simulink model "PumpSeries_linearOrQuadraticCharacter"  (R2018b)
settings: Solver=ode45  StartTime=0.0  StopTime=100  MaxStep=5  RelTol=1e-3  EnableMultiTasking=on
undefined symbols (not defined in the file): DiameterLastPiece, DPConstant, DPLinear, DPQuadratic, ID, MassFlow, path_carnot, Pressure, Temperature, Water
libraries: carnot x15, simulink x3
settings Model: EnablePacing=on  Creator=drhf  LastModifiedBy=drhf
settings DataIOCC: SaveFormat=Array  SignalLoggingSaveFormat=ModelDataLogs
settings OptimizationCC: ExpressionDepthLimit=2147483647  LifeSpan=inf
settings DebuggingCC: UnderspecifiedInitializationDetection=Classic  MergeDetectMultiDrivingBlocksExec=none  SolverPrmCheckMsg=warning  StateNameClashWarn=warning  SFUnexpectedBacktrackingDiag=warning  SFNoUnconditionalDefaultTransitionDiag=warning  SFExecutionAtInitializationDiag=none
settings HardwareCC: ProdBitPerPointer=32  ProdBitPerSizeT=32  ProdBitPerPtrDiffT=32  ProdLargestAtomicFloat=None  ProdIntDivRoundTo=Undefined  ProdEndianess=Unspecified  ProdWordSize=32  ProdHWDeviceType=32-bit Generic
settings ModelReferenceCC: PropagateSignalLabelsOutOfModel=off
settings SFSimCC: SimUseLocalCustomCode=off
settings RTWCC: RTWUseLocalCustomCode=off
settings CodeAppCC: StateflowObjectComments=on
settings GRTTargetCC: TargetLangStandard=C89/C90 (ANSI)  GeneratePreprocessorConditionals=Disable all  CombineOutputUpdateFcns=off  GRTInterface=on
settings ConfigComp: CovMetricSettings=dw  CovHtmlReporting=on  CovSaveCumulativeToWorkspaceVar=on  CovSaveSingleToWorkspaceVar=on  CovExternalEMLEnable=off

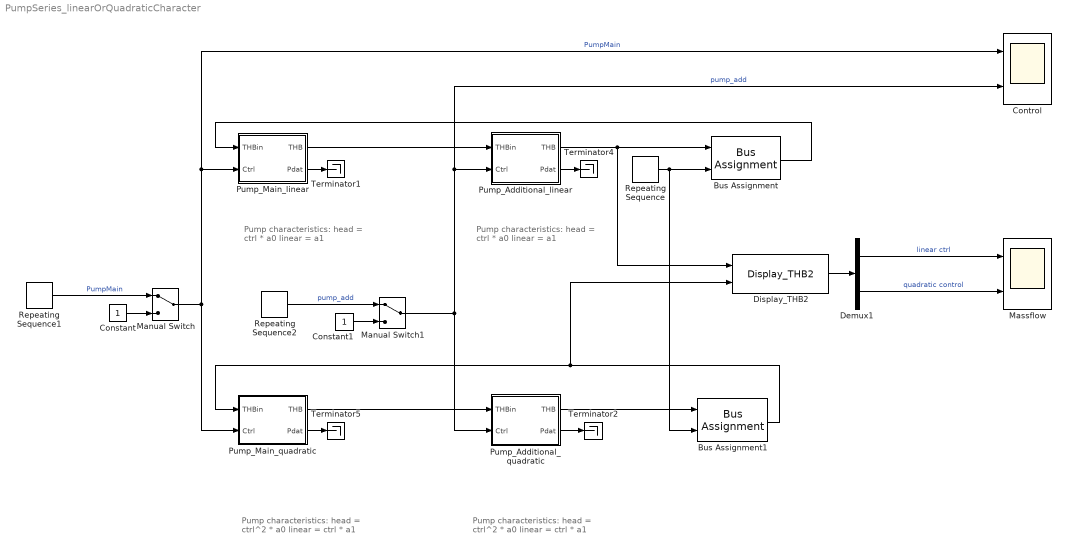
== system PumpSeries_linearOrQuadraticCharacter ==
  note: Pump characteristics:
      | head = ctrl^2 * a0
      | linear = ctrl * a1
  note: Pump characteristics:
      | head = ctrl * a0
      | linear = a1
  note: Pump characteristics:
      | head = ctrl * a0
      | linear = a1
  note: Pump characteristics:
      | head = ctrl^2 * a0
      | linear = ctrl * a1
  Bus Assignment : BusAssignment  AssignedSignals=DPQuadratic
  Bus Assignment1 : BusAssignment  AssignedSignals=DPQuadratic
  Constant : Constant
  Constant1 : Constant
  Control : Scope  NumInputPorts=2
  Demux1 : Demux  Outputs=2
  Display_THB2 : carnot/Outputs/Display_THB2  t=off  m=on  p=off  id=off  mix=off  d=off
      settings: SourceProductName=Carnot
  Manual Switch : ManualSwitch
  Manual Switch1 : ManualSwitch
  Massflow : Scope  NumInputPorts=2
  Pump_Additional_linear : Subsystem  AncestorBlock=carnot/Hydraulics/Pump_Additional  mask(Pump Additional){Tini=20, PathName=fullfile(path_carnot('libsl'), 'Hydraulics', 'Pump_Main', 'parameter_set'), FileName='Pump6m.mat', userPath=off, userParam=off, a0=60000, a1=-43200, a2=0, dia=0.025, UA=1, mcp=4182, e0=50, e1=28.8, e2=-10.368}
      mask prompts: Tini "Ambient temperature for losses and initial temperture in °C"; PathName "Path"; FileName "Parameter set"; userPath "Edit path and name of parameter set"; userParam "User defined parameters"; a0 "a0: pump head in [Pa] (pressure increase at zero flow)"; a1 "a1: pump characteristic linear coefficient [Pa*s/kg]"; a2 "a2: pump characteristic quadratic coefficient [Pa*(s/kg)²]"; dia "Diameter at in- and outlet [m]"; UA "UA: thermal loss coefficient in W/K"; mcp "mcp: thermal capacity of the node in J/K"; e0 "e0: constant coefficient in W"; e1 "e1: linear coefficient in W*s/kg"; e2 "e2: quadratic coefficient in W*(s/kg)²"
      mask help:
      | This is an additional pump in a circuit. Every circuit must have exactly ONE 'Pump_Main'. It may have several 'Pump_Additional' blocks. The pump adds pump_head to the pressure drop of the circuit dp_circuit:
      |     dp_circuit = c + l*mdot + q*(mdot)²
      |     pump_head_ = a0*Ctrl² + a1*Ctrl*mdot +a2*mdot²
      |     dp_total = pump_head - dp_circuit
      |     p1 = system_pressure + (a0*Ctrl² - c) + (a1*Ctrl - l) * mdot + (a2-q)*(mdot)²
      | with
      |   Ctrl : Control signal input [0..1]
      | Note: Pump_Additional uses the parameters sets as Pump_Main.
      mask init:
      | % callback to set parameters of model
      | [ok, param] = CarnotCallbacks_PumpAdditional('SetParameters',gcbh,PathName,FileName);
      mask Help: web(fullfile(path_carnot('help'),'Pump_Main.html'),'-helpbrowser')
      mask TypeOptions Tini: ThermalNodeTHB/Tini
      mask Callback userPath: [ok, param] = CarnotCallbacks_PumpAdditional('UserEdit',gcbh);
      mask Callback userParam: [ok, param] = CarnotCallbacks_PumpAdditional('UserEdit',gcbh);
      mask TypeOptions a0: PumpHead/Gain
      mask TypeOptions a1: PumpLinear/Gain
      mask TypeOptions a2: PumpQuadratic/Value
      mask TypeOptions dia: dia/Value
      mask TypeOptions UA: ThermalNodeTHB/UA
      mask TypeOptions mcp: ThermalNodeTHB/mcp
      mask TypeOptions e0: ElectricConsumptionPump/e0
      mask TypeOptions e1: ElectricConsumptionPump/e1
      mask TypeOptions e2: ElectricConsumptionPump/e2
      mask DialogControl ParameterGroupFile Prompt: Picking a parameter set
      mask DialogControl Control1 Prompt: Carnot public data
      mask DialogControl Control1 Callback: [ok, file] = CarnotCallbacks_PumpAdditional('GetFilename',gcbh,'public');
      mask DialogControl Control3 Prompt: Carnot internal data
      mask DialogControl Control3 Callback: [ok, file] = CarnotCallbacks_PumpAdditional('GetFilename',gcbh,'internal');
      mask DialogControl Control4 Prompt: Selected path
      mask DialogControl Control4 Callback: [ok, file] = CarnotCallbacks_PumpAdditional('GetFilename',gcbh,'selected');
      mask DialogControl PrameterGroupUser Prompt: Parameter Values
      mask DialogControl Container9 Prompt: Hydraulic
      mask DialogControl Container7 Prompt: Thermal
      mask DialogControl Control9 Prompt: Thermal node for temperature:  mcp * dTnode/dt = UA*(Tamb-Tnode) + mdot*cp_in*(Tin-Tnode)
      mask DialogControl Container12 Prompt: Electric
      mask DialogControl Control7 Prompt: Power consumption  Pel = e0 + e1*mdot + e2*mdot²
      mask DialogControl Control5 Prompt: Save in Carnot internal data
      mask DialogControl Control5 Callback: [ok, param] = CarnotCallbacks_PumpAdditional('SaveFilename',gcbh,'internal','B');
      mask DialogControl Control6 Prompt: Save in selected path
      mask DialogControl Control6 Callback: [ok, param] = CarnotCallbacks_PumpAdditional('SaveFilename',gcbh,'selected','B');
      mask Display:
      | % user defined picture file
      | picfile = fullfile(path_carnot('intlibsl'), ...
      |         'Hydraulics', 'Pump_Additional', 'PumpAdditional.jpg');
      | 
      | pic = false;
      | if ~BlockIsInCarnotLibrary    % if not located in library any more
      |     if exist(picfile,'file') % show internal picture if defined
      |         image(imread(picfile), [0.2, 0, 0.6, 1])
      |         set_param(gcb, 'BackgroundColor', 'White')
      |         pic = true;
      |     end
      | end
      | if ~pic    % show public picture
      |     set_param(gcb, 'BackgroundColor', 'green')
      |     plot(0,0,1,1,[40,70,40,30,30,40,60,70,70,60,40]/100, ...
      |         [70,50,30,40,60,70,70,60,40,30,30]/100)
      |     disp('add')
      | end
  Pump_Additional_quadratic : Subsystem  AncestorBlock=carnot/Hydraulics/Pump_Additional  mask(Pump Additional){Tini=20, PathName=fullfile(path_carnot('libsl'), 'Hydraulics', 'Pump_Main', 'parameter_set'), FileName='Pump6m.mat', userPath=off, userParam=off, a0=60000, a1=-43200, a2=0, dia=0.025, UA=1, mcp=4182, e0=50, e1=28.8, e2=-10.368}
      mask prompts: Tini "Ambient temperature for losses and initial temperture in °C"; PathName "Path"; FileName "Parameter set"; userPath "Edit path and name of parameter set"; userParam "User defined parameters"; a0 "a0: pump head in [Pa] (pressure increase at zero flow)"; a1 "a1: pump characteristic linear coefficient [Pa*s/kg]"; a2 "a2: pump characteristic quadratic coefficient [Pa*(s/kg)²]"; dia "Diameter at in- and outlet [m]"; UA "UA: thermal loss coefficient in W/K"; mcp "mcp: thermal capacity of the node in J/K"; e0 "e0: constant coefficient in W"; e1 "e1: linear coefficient in W*s/kg"; e2 "e2: quadratic coefficient in W*(s/kg)²"
      mask help:
      | This is an additional pump in a circuit. Every circuit must have exactly ONE 'Pump_Main'. It may have several 'Pump_Additional' blocks. The pump adds pump_head to the pressure drop of the circuit dp_circuit:
      |     dp_circuit = c + l*mdot + q*(mdot)²
      |     pump_head_ = a0*Ctrl² + a1*Ctrl*mdot +a2*mdot²
      |     dp_total = pump_head - dp_circuit
      |     p1 = system_pressure + (a0*Ctrl² - c) + (a1*Ctrl - l) * mdot + (a2-q)*(mdot)²
      | with
      |   Ctrl : Control signal input [0..1]
      | Note: Pump_Additional uses the parameters sets as Pump_Main.
      mask init:
      | % callback to set parameters of model
      | [ok, param] = CarnotCallbacks_PumpAdditional('SetParameters',gcbh,PathName,FileName);
      mask Help: web(fullfile(path_carnot('help'),'Pump_Main.html'),'-helpbrowser')
      mask TypeOptions Tini: ThermalNodeTHB/Tini
      mask Callback userPath: [ok, param] = CarnotCallbacks_PumpAdditional('UserEdit',gcbh);
      mask Callback userParam: [ok, param] = CarnotCallbacks_PumpAdditional('UserEdit',gcbh);
      mask TypeOptions a0: PumpHead/Gain
      mask TypeOptions a1: PumpLinear/Gain
      mask TypeOptions a2: PumpQuadratic/Value
      mask TypeOptions dia: dia/Value
      mask TypeOptions UA: ThermalNodeTHB/UA
      mask TypeOptions mcp: ThermalNodeTHB/mcp
      mask TypeOptions e0: ElectricConsumptionPump/e0
      mask TypeOptions e1: ElectricConsumptionPump/e1
      mask TypeOptions e2: ElectricConsumptionPump/e2
      mask DialogControl ParameterGroupFile Prompt: Picking a parameter set
      mask DialogControl Control1 Prompt: Carnot public data
      mask DialogControl Control1 Callback: [ok, file] = CarnotCallbacks_PumpAdditional('GetFilename',gcbh,'public');
      mask DialogControl Control3 Prompt: Carnot internal data
      mask DialogControl Control3 Callback: [ok, file] = CarnotCallbacks_PumpAdditional('GetFilename',gcbh,'internal');
      mask DialogControl Control4 Prompt: Selected path
      mask DialogControl Control4 Callback: [ok, file] = CarnotCallbacks_PumpAdditional('GetFilename',gcbh,'selected');
      mask DialogControl PrameterGroupUser Prompt: Parameter Values
      mask DialogControl Container9 Prompt: Hydraulic
      mask DialogControl Container7 Prompt: Thermal
      mask DialogControl Control9 Prompt: Thermal node for temperature:  mcp * dTnode/dt = UA*(Tamb-Tnode) + mdot*cp_in*(Tin-Tnode)
      mask DialogControl Container12 Prompt: Electric
      mask DialogControl Control7 Prompt: Power consumption  Pel = e0 + e1*mdot + e2*mdot²
      mask DialogControl Control5 Prompt: Save in Carnot internal data
      mask DialogControl Control5 Callback: [ok, param] = CarnotCallbacks_PumpAdditional('SaveFilename',gcbh,'internal','B');
      mask DialogControl Control6 Prompt: Save in selected path
      mask DialogControl Control6 Callback: [ok, param] = CarnotCallbacks_PumpAdditional('SaveFilename',gcbh,'selected','B');
      mask Display:
      | % user defined picture file
      | picfile = fullfile(path_carnot('intlibsl'), ...
      |         'Hydraulics', 'Pump_Additional', 'PumpAdditional.jpg');
      | 
      | pic = false;
      | if ~BlockIsInCarnotLibrary    % if not located in library any more
      |     if exist(picfile,'file') % show internal picture if defined
      |         image(imread(picfile), [0.2, 0, 0.6, 1])
      |         set_param(gcb, 'BackgroundColor', 'White')
      |         pic = true;
      |     end
      | end
      | if ~pic    % show public picture
      |     set_param(gcb, 'BackgroundColor', 'green')
      |     plot(0,0,1,1,[40,70,40,30,30,40,60,70,70,60,40]/100, ...
      |         [70,50,30,40,60,70,70,60,40,30,30]/100)
      |     disp('add')
      | end
  Pump_Main_linear : Subsystem  AncestorBlock=carnot/Hydraulics/Pump_Main  mask(Pump Main){Tini=20, p0=3e5, IDpreset=pressure drop, fluid=Water, mix=0, mix2=0, mix3=0, t1=1, PathName=fullfile(path_carnot('libsl'), 'Hydraulics', 'Pump_Main', 'parameter_set'), FileName='Pump6m.mat', userPath=off, userParam=off, a0=60000, a1=-43200, a2=0, dia=0.025, UA=1, mcp=4182, e0=50, e1=28.8, e2=-10.368}
      mask prompts: Tini "Ambient temperature for losses and initial temperture in °C"; p0 "System pressure at pump inlet [Pa]"; IDpreset "Pressure calculation"; mix "Fluid mixture    [0..1]"; mix2 "Fluid mixture 2 [0..1]"; mix3 "Fluid mixture 3 [0..1]"; t1 "Time constant [s] of pump"; PathName "Path"; FileName "Parameter set"; userPath "Edit path and name of parameter set"; userParam "User defined parameters"; a0 "a0: pump head in [Pa] (pressure increase at zero flow)"; a1 "a1: pump characteristic linear coefficient [Pa*s/kg]"; a2 "a2: pump characteristic quadratic coefficient [Pa*(s/kg)²]"; dia "Diameter at in- and outlet [m]"; UA "UA: thermal loss coefficient in W/K"; mcp "mcp: thermal capacity of the node in J/K"; e0 "e0: constant coefficient in W"; e1 "e1: linear coefficient in W*s/kg"; e2 "e2: quadratic coefficient in W*(s/kg)²"
      mask help:
      | This is the main pump in a circuit. Every circuit must have exactly ONE 'Pump_Main'. Use the 'Pump_Additional' blocks if you want to use more pumps.
      | The Pump_Main calculate massflow by setting pressure drop in the circuit (dp_circuit) equal to the pressure increase of the pump (pump_head).
      |   dp_circuit = c + l*mdot + q*mdot²
      |   pump_head_ = a0*Ctrl² + a1*Ctrl*mdot +a2*mdot²
      | with
      |   mdot : massflow in kg/s
      |   Ctrl : Control signal input [0..1]
      | This model uses a Memory block to break an algebraic loop. Avoid using the variable-step solver ode15s or ode113 (see block help for details).
      | A unit delay block with a sample time ("time constant of the pump") limits the maximum stepsize.
      mask init:
      | % callback to set parameters of model
      | [ok, param] = CarnotCallbacks_PumpMain('SetParameters',gcbh,PathName,FileName);
      mask Help: web(fullfile(path_carnot('help'),'Pump_Main.html'),'-helpbrowser')
      mask TypeOptions Tini: ThermalNodeTHB/Tini
      mask TypeOptions p0: basic_THB/p
      mask TypeOptions IDpreset: ID/IDpreset
      mask TypeOptions fluid: basic_THB/fluid
      mask TypeOptions mix: basic_THB/mix
      mask TypeOptions mix2: basic_THB/mix2
      mask TypeOptions mix3: basic_THB/mix3
      mask TypeOptions t1: UnitDelay/SampleTime
      mask Callback userPath: [ok, param] = CarnotCallbacks_PumpMain('UserEdit',gcbh);
      mask Callback userParam: [ok, param] = CarnotCallbacks_PumpMain('UserEdit',gcbh);
      mask TypeOptions a0: PumpHead/Gain
      mask TypeOptions a1: PumpLinear/Value
      mask TypeOptions a2: PumpQuadratic/Value
      mask TypeOptions dia: basic_THB/dia
      mask TypeOptions UA: ThermalNodeTHB/UA
      mask TypeOptions mcp: ThermalNodeTHB/mcp
      mask TypeOptions e0: ElectricConsumptionPump/e0
      mask TypeOptions e1: ElectricConsumptionPump/e1
      mask TypeOptions e2: ElectricConsumptionPump/e2
      mask DialogControl ParameterGroupFile Prompt: Picking a parameter set
      mask DialogControl Control1 Prompt: Carnot public data
      mask DialogControl Control1 Callback: [ok, file] = CarnotCallbacks_PumpMain('GetFilename',gcbh,'public');
      mask DialogControl Control3 Prompt: Carnot internal data
      mask DialogControl Control3 Callback: [ok, file] = CarnotCallbacks_PumpMain('GetFilename',gcbh,'internal');
      mask DialogControl Control4 Prompt: Selected path
      mask DialogControl Control4 Callback: [ok, file] = CarnotCallbacks_PumpMain('GetFilename',gcbh,'selected');
      mask DialogControl PrameterGroupUser Prompt: Parameter Values
      mask DialogControl Container9 Prompt: Hydraulic
      mask DialogControl Container7 Prompt: Thermal
      mask DialogControl Control9 Prompt: Thermal node for temperature:  mcp * dTnode/dt = UA*(Tamb-Tnode) + mdot*cp_in*(Tin-Tnode)
      mask DialogControl Container14 Prompt: Electric
      mask DialogControl Control7 Prompt: Power consumption  Pel = e0 + e1*mdot + e2*mdot²
      mask DialogControl Control5 Prompt: Save in Carnot internal data
      mask DialogControl Control5 Callback: [ok, param] = CarnotCallbacks_PumpMain('SaveFilename',gcbh,'internal','B');
      mask DialogControl Control6 Prompt: Save in selected path
      mask DialogControl Control6 Callback: [ok, param] = CarnotCallbacks_PumpMain('SaveFilename',gcbh,'selected','B');
      mask Display:
      | % user defined picture file
      | picfile = fullfile(path_carnot('intlibsl'), ...
      |         'Hydraulics', 'Pump_Main', 'PumpMain.jpg');
      | 
      | pic = false;
      | if ~BlockIsInCarnotLibrary    % if not located in library any more
      |     if exist(picfile,'file') % show internal picture if defined
      |         image(imread(picfile), [0.2, 0, 0.6, 1])
      |         set_param(gcb, 'BackgroundColor', 'White')
      |         pic = true;
      |     end
      | end
      | if ~pic    % show public picture
      |     set_param(gcb, 'BackgroundColor', 'green')
      |     plot(0,0,1,1,[40,70,40,30,30,40,60,70,70,60,40]/100, ...
      |         [70,50,30,40,60,70,70,60,40,30,30]/100)
      |     disp('main')
      | end
  Pump_Main_quadratic : Subsystem  AncestorBlock=carnot/Hydraulics/Pump_Main  mask(Pump Main){Tini=20, p0=3e5, IDpreset=pressure drop, fluid=Water, mix=0, mix2=0, mix3=0, t1=1, PathName=fullfile(path_carnot('libsl'), 'Hydraulics', 'Pump_Main', 'parameter_set'), FileName='Pump6m.mat', userPath=off, userParam=off, a0=60000, a1=-43200, a2=0, dia=0.025, UA=1, mcp=4182, e0=50, e1=28.8, e2=-10.368}
      mask prompts: Tini "Ambient temperature for losses and initial temperture in °C"; p0 "System pressure at pump inlet [Pa]"; IDpreset "Pressure calculation"; mix "Fluid mixture    [0..1]"; mix2 "Fluid mixture 2 [0..1]"; mix3 "Fluid mixture 3 [0..1]"; t1 "Time constant [s] of pump"; PathName "Path"; FileName "Parameter set"; userPath "Edit path and name of parameter set"; userParam "User defined parameters"; a0 "a0: pump head in [Pa] (pressure increase at zero flow)"; a1 "a1: pump characteristic linear coefficient [Pa*s/kg]"; a2 "a2: pump characteristic quadratic coefficient [Pa*(s/kg)²]"; dia "Diameter at in- and outlet [m]"; UA "UA: thermal loss coefficient in W/K"; mcp "mcp: thermal capacity of the node in J/K"; e0 "e0: constant coefficient in W"; e1 "e1: linear coefficient in W*s/kg"; e2 "e2: quadratic coefficient in W*(s/kg)²"
      mask help:
      | This is the main pump in a circuit. Every circuit must have exactly ONE 'Pump_Main'. Use the 'Pump_Additional' blocks if you want to use more pumps.
      | The Pump_Main calculate massflow by setting pressure drop in the circuit (dp_circuit) equal to the pressure increase of the pump (pump_head).
      |   dp_circuit = c + l*mdot + q*mdot²
      |   pump_head_ = a0*Ctrl² + a1*Ctrl*mdot +a2*mdot²
      | with
      |   mdot : massflow in kg/s
      |   Ctrl : Control signal input [0..1]
      | This model uses a Memory block to break an algebraic loop. Avoid using the variable-step solver ode15s or ode113 (see block help for details).
      | A unit delay block with a sample time ("time constant of the pump") limits the maximum stepsize.
      mask init:
      | % callback to set parameters of model
      | [ok, param] = CarnotCallbacks_PumpMain('SetParameters',gcbh,PathName,FileName);
      mask Help: web(fullfile(path_carnot('help'),'Pump_Main.html'),'-helpbrowser')
      mask TypeOptions Tini: ThermalNodeTHB/Tini
      mask TypeOptions p0: basic_THB/p
      mask TypeOptions IDpreset: ID/IDpreset
      mask TypeOptions fluid: basic_THB/fluid
      mask TypeOptions mix: basic_THB/mix
      mask TypeOptions mix2: basic_THB/mix2
      mask TypeOptions mix3: basic_THB/mix3
      mask TypeOptions t1: UnitDelay/SampleTime
      mask Callback userPath: [ok, param] = CarnotCallbacks_PumpMain('UserEdit',gcbh);
      mask Callback userParam: [ok, param] = CarnotCallbacks_PumpMain('UserEdit',gcbh);
      mask TypeOptions a0: PumpHead/Gain
      mask TypeOptions a1: PumpLinear/Value
      mask TypeOptions a2: PumpQuadratic/Value
      mask TypeOptions dia: basic_THB/dia
      mask TypeOptions UA: ThermalNodeTHB/UA
      mask TypeOptions mcp: ThermalNodeTHB/mcp
      mask TypeOptions e0: ElectricConsumptionPump/e0
      mask TypeOptions e1: ElectricConsumptionPump/e1
      mask TypeOptions e2: ElectricConsumptionPump/e2
      mask DialogControl ParameterGroupFile Prompt: Picking a parameter set
      mask DialogControl Control1 Prompt: Carnot public data
      mask DialogControl Control1 Callback: [ok, file] = CarnotCallbacks_PumpMain('GetFilename',gcbh,'public');
      mask DialogControl Control3 Prompt: Carnot internal data
      mask DialogControl Control3 Callback: [ok, file] = CarnotCallbacks_PumpMain('GetFilename',gcbh,'internal');
      mask DialogControl Control4 Prompt: Selected path
      mask DialogControl Control4 Callback: [ok, file] = CarnotCallbacks_PumpMain('GetFilename',gcbh,'selected');
      mask DialogControl PrameterGroupUser Prompt: Parameter Values
      mask DialogControl Container9 Prompt: Hydraulic
      mask DialogControl Container7 Prompt: Thermal
      mask DialogControl Control9 Prompt: Thermal node for temperature:  mcp * dTnode/dt = UA*(Tamb-Tnode) + mdot*cp_in*(Tin-Tnode)
      mask DialogControl Container14 Prompt: Electric
      mask DialogControl Control7 Prompt: Power consumption  Pel = e0 + e1*mdot + e2*mdot²
      mask DialogControl Control5 Prompt: Save in Carnot internal data
      mask DialogControl Control5 Callback: [ok, param] = CarnotCallbacks_PumpMain('SaveFilename',gcbh,'internal','B');
      mask DialogControl Control6 Prompt: Save in selected path
      mask DialogControl Control6 Callback: [ok, param] = CarnotCallbacks_PumpMain('SaveFilename',gcbh,'selected','B');
      mask Display:
      | % user defined picture file
      | picfile = fullfile(path_carnot('intlibsl'), ...
      |         'Hydraulics', 'Pump_Main', 'PumpMain.jpg');
      | 
      | pic = false;
      | if ~BlockIsInCarnotLibrary    % if not located in library any more
      |     if exist(picfile,'file') % show internal picture if defined
      |         image(imread(picfile), [0.2, 0, 0.6, 1])
      |         set_param(gcb, 'BackgroundColor', 'White')
      |         pic = true;
      |     end
      | end
      | if ~pic    % show public picture
      |     set_param(gcb, 'BackgroundColor', 'green')
      |     plot(0,0,1,1,[40,70,40,30,30,40,60,70,70,60,40]/100, ...
      |         [70,50,30,40,60,70,70,60,40,30,30]/100)
      |     disp('main')
      | end
  Repeating Sequence : simulink/Sources/Repeating Sequence  rep_seq_t=[0 200 200.1 400]  rep_seq_y="0*[1 1 1 1]*1e4   %[0 0 1 1]*(6e4/0.01)^2"
  Repeating Sequence1 : simulink/Sources/Repeating Sequence  rep_seq_t=[0 40 50 60 70 100]  rep_seq_y=[1 1 0 0 1 1]
  Repeating Sequence2 : simulink/Sources/Repeating Sequence  rep_seq_t=[0 5 20 100]  rep_seq_y=[0 0 1 1]
  Terminator{1..2,4..5} (4 alike) : Terminator
  wires:
  Pump_Additional_quadratic/2(Pdat) -> Terminator2/1
  Manual Switch/1 -> Pump_Main_linear/2(Ctrl), Control/1, Pump_Main_quadratic/2(Ctrl)  "PumpMain"
  Bus Assignment/1 -> Pump_Main_linear/1(THBin)
  Pump_Main_linear/2(Pdat) -> Terminator1/1
  Repeating Sequence/1 -> Bus Assignment1/2, Bus Assignment/2
  Pump_Main_linear/1(THB) -> Pump_Additional_linear/1(THBin)
  Display_THB2/1 -> Demux1/1
  Pump_Additional_linear/2(Pdat) -> Terminator4/1
  Manual Switch1/1 -> Pump_Additional_quadratic/2(Ctrl), Control/2, Pump_Additional_linear/2(Ctrl)  "pump_add"
  Demux1/1 -> Massflow/1  "linear ctrl"
  Demux1/2 -> Massflow/2  "quadratic control"
  Pump_Additional_linear/1(THB) -> Bus Assignment/1, Display_THB2/1
  Repeating Sequence1/1 -> Manual Switch/1  "PumpMain"
  Constant/1 -> Manual Switch/2
  Constant1/1 -> Manual Switch1/2
  Repeating Sequence2/1 -> Manual Switch1/1  "pump_add"
  Bus Assignment1/1 -> Display_THB2/2, Pump_Main_quadratic/1(THBin)
  Pump_Main_quadratic/1(THB) -> Pump_Additional_quadratic/1(THBin)
  Pump_Main_quadratic/2(Pdat) -> Terminator5/1
  Pump_Additional_quadratic/1(THB) -> Bus Assignment1/1

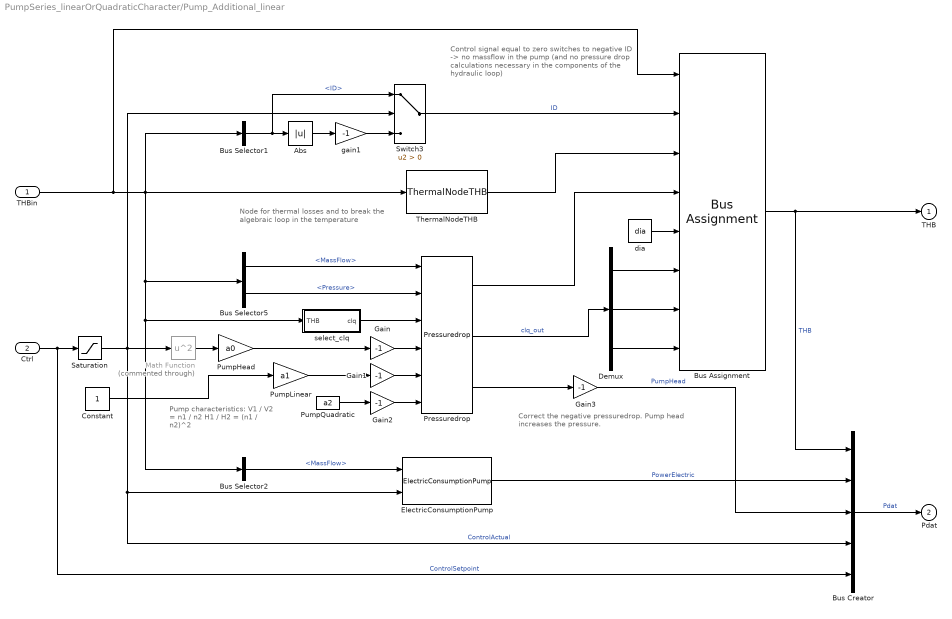
== system PumpSeries_linearOrQuadraticCharacter/Pump_Additional_linear ==
  note: Node for thermal losses and to break
      | the algebraic loop in the temperature
  note: Control signal equal to zero switches
      | to negative ID -> no massflow in the
      | pump (and no pressure drop calculations
      | necessary in the components of the
      | hydraulic loop)
  note: Correct the negative pressuredrop.
      | Pump head increases the pressure.
  note: Pump characteristics:
      | V1 / V2 = n1 / n2
      | H1 / H2 = (n1 / n2)^2
  THBin : Inport
  Ctrl : Inport  Port=2
  Abs : Abs
  Bus Assignment : BusAssignment  AssignedSignals=ID,Temperature,Pressure,DiameterLastPiece,DPConstant,DPLinear,DPQuadratic
  Bus Creator : BusCreator  Inputs=5
  Bus Selector1 : BusSelector  OutputSignals=ID
  Bus Selector2 : BusSelector  OutputSignals=MassFlow
  Bus Selector5 : BusSelector  OutputSignals=MassFlow,Pressure
  Constant : Constant
  Demux : Demux  Outputs=3
  ElectricConsumptionPump : carnot/Basic/Hydraulics/ElectricConsumptionPump  e0=e0  e1=e1  e2=e2
      settings: SourceProductName=Carnot
  Gain{,1..3} (4 alike) : Gain  Gain=-1
  Math Function : Math  Commented=through  Operator=square  SaturateOnIntegerOverflow=on
  Pressuredrop : carnot/Basic/Pressure_Drop/Pressuredrop
      settings: SourceProductName=Carnot
  PumpHead : Gain  Gain=a0
  PumpLinear : Gain  Gain=a1
  PumpQuadratic : Constant  Value=a2
  Saturation : Saturate  UpperLimit=1  LowerLimit=0
  Switch3 : Switch  Criteria=u2 > Threshold  SaturateOnIntegerOverflow=on  InputSameDT=on
  ThermalNodeTHB : carnot/Basic/Thermal_Models/ThermalNodeTHB  UA=UA  mcp=mcp  Tini=Tini
      settings: SourceProductName=Carnot
  dia : Constant  Value=dia
  gain1 : Gain  Gain=-1  SaturateOnIntegerOverflow=on  OutDataTypeStr=Inherit: Same as input  ParamDataTypeStr=Inherit: Same as input
  select_clq : Subsystem
  THB : Outport
  Pdat : Outport  Port=2
  wires:
  Gain2/1 -> Pressuredrop/6
  Gain1/1 -> Pressuredrop/5
  Gain/1 -> Pressuredrop/4
  Bus Selector5/2 -> Pressuredrop/2  "<Pressure>"
  select_clq/1(clq) -> Pressuredrop/3
  ThermalNodeTHB/1 -> Bus Assignment/3
  Demux/3 -> Bus Assignment/8
  Demux/2 -> Bus Assignment/7
  Demux/1 -> Bus Assignment/6
  PumpQuadratic/1 -> Gain2/1
  PumpLinear/1 -> Gain1/1
  PumpHead/1 -> Gain/1
  THBin/1 -> Bus Assignment/1, ThermalNodeTHB/1, Bus Selector5/1, select_clq/1(THB), Bus Selector2/1, Bus Selector1/1
  dia/1 -> Bus Assignment/5
  Bus Selector5/1 -> Pressuredrop/1  "<MassFlow>"
  Switch3/1 -> Bus Assignment/2  "ID"
  gain1/1 -> Switch3/3
  Abs/1 -> gain1/1
  Bus Selector1/1 -> Abs/1, Switch3/1  "<ID>"
  Ctrl/1 -> Bus Creator/5, Saturation/1  "ControlSetpoint"
  ElectricConsumptionPump/1 -> Bus Creator/2  "PowerElectric"
  Bus Creator/1 -> Pdat/1  "Pdat"
  Bus Selector2/1 -> ElectricConsumptionPump/1  "<MassFlow>"
  Bus Assignment/1 -> Bus Creator/1, THB/1  "THB"
  Pressuredrop/3 -> Gain3/1
  Pressuredrop/2 -> Demux/1  "clq_out"
  Pressuredrop/1 -> Bus Assignment/4
  Gain3/1 -> Bus Creator/3  "PumpHead"
  Saturation/1 -> Math Function/1, ElectricConsumptionPump/2, Bus Creator/4, Switch3/2  "ControlActual"
  Math Function/1 -> PumpHead/1
  Constant/1 -> PumpLinear/1

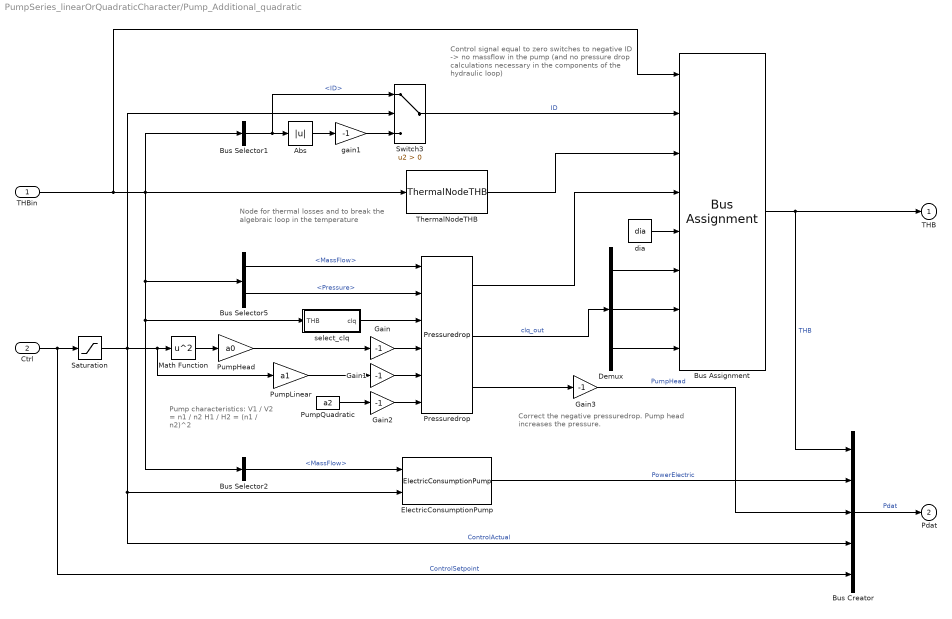
== system PumpSeries_linearOrQuadraticCharacter/Pump_Additional_quadratic ==
  note: Pump characteristics:
      | V1 / V2 = n1 / n2
      | H1 / H2 = (n1 / n2)^2
  note: Correct the negative pressuredrop.
      | Pump head increases the pressure.
  note: Control signal equal to zero switches
      | to negative ID -> no massflow in the
      | pump (and no pressure drop calculations
      | necessary in the components of the
      | hydraulic loop)
  note: Node for thermal losses and to break
      | the algebraic loop in the temperature
  THBin : Inport
  Ctrl : Inport  Port=2
  Abs : Abs
  Bus Assignment : BusAssignment  AssignedSignals=ID,Temperature,Pressure,DiameterLastPiece,DPConstant,DPLinear,DPQuadratic
  Bus Creator : BusCreator  Inputs=5
  Bus Selector1 : BusSelector  OutputSignals=ID
  Bus Selector2 : BusSelector  OutputSignals=MassFlow
  Bus Selector5 : BusSelector  OutputSignals=MassFlow,Pressure
  Demux : Demux  Outputs=3
  ElectricConsumptionPump : carnot/Basic/Hydraulics/ElectricConsumptionPump  e0=e0  e1=e1  e2=e2
      settings: SourceProductName=Carnot
  Gain{,1..3} (4 alike) : Gain  Gain=-1
  Math Function : Math  Operator=square  SaturateOnIntegerOverflow=on
  Pressuredrop : carnot/Basic/Pressure_Drop/Pressuredrop
      settings: SourceProductName=Carnot
  PumpHead : Gain  Gain=a0
  PumpLinear : Gain  Gain=a1
  PumpQuadratic : Constant  Value=a2
  Saturation : Saturate  UpperLimit=1  LowerLimit=0
  Switch3 : Switch  Criteria=u2 > Threshold  SaturateOnIntegerOverflow=on  InputSameDT=on
  ThermalNodeTHB : carnot/Basic/Thermal_Models/ThermalNodeTHB  UA=UA  mcp=mcp  Tini=Tini
      settings: SourceProductName=Carnot
  dia : Constant  Value=dia
  gain1 : Gain  Gain=-1  SaturateOnIntegerOverflow=on  OutDataTypeStr=Inherit: Same as input  ParamDataTypeStr=Inherit: Same as input
  select_clq : Subsystem
  THB : Outport
  Pdat : Outport  Port=2
  wires:
  Math Function/1 -> PumpHead/1
  Saturation/1 -> Switch3/2, Bus Creator/4, ElectricConsumptionPump/2, PumpLinear/1, Math Function/1  "ControlActual"
  Gain3/1 -> Bus Creator/3  "PumpHead"
  Pressuredrop/1 -> Bus Assignment/4
  Pressuredrop/2 -> Demux/1  "clq_out"
  Pressuredrop/3 -> Gain3/1
  Bus Assignment/1 -> THB/1, Bus Creator/1  "THB"
  Bus Selector2/1 -> ElectricConsumptionPump/1  "<MassFlow>"
  Bus Creator/1 -> Pdat/1  "Pdat"
  ElectricConsumptionPump/1 -> Bus Creator/2  "PowerElectric"
  Ctrl/1 -> Saturation/1, Bus Creator/5  "ControlSetpoint"
  Bus Selector1/1 -> Switch3/1, Abs/1  "<ID>"
  Abs/1 -> gain1/1
  gain1/1 -> Switch3/3
  Switch3/1 -> Bus Assignment/2  "ID"
  Bus Selector5/1 -> Pressuredrop/1  "<MassFlow>"
  dia/1 -> Bus Assignment/5
  THBin/1 -> Bus Selector1/1, Bus Selector2/1, select_clq/1(THB), Bus Selector5/1, ThermalNodeTHB/1, Bus Assignment/1
  PumpHead/1 -> Gain/1
  PumpLinear/1 -> Gain1/1
  PumpQuadratic/1 -> Gain2/1
  Demux/1 -> Bus Assignment/6
  Demux/2 -> Bus Assignment/7
  Demux/3 -> Bus Assignment/8
  ThermalNodeTHB/1 -> Bus Assignment/3
  select_clq/1(clq) -> Pressuredrop/3
  Bus Selector5/2 -> Pressuredrop/2  "<Pressure>"
  Gain/1 -> Pressuredrop/4
  Gain1/1 -> Pressuredrop/5
  Gain2/1 -> Pressuredrop/6

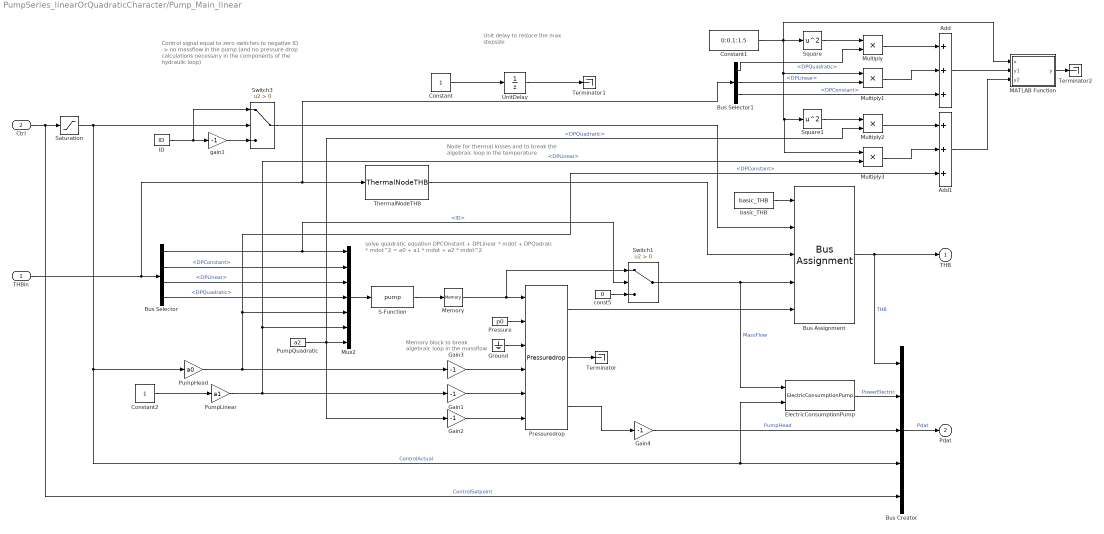
== system PumpSeries_linearOrQuadraticCharacter/Pump_Main_linear ==
  note: Node for thermal losses and to break
      | the algebraic loop in the temperature
  note: Memory block to
      | break algebraic loop
      | in the massflow
  note: solve quadratic equation
      | DPCOnstant + DPLinear * mdot + DPQadraic * mdot^2
      | = a0 + a1 * mdot + a2 * mdot^2
  note: Control signal equal to zero switches
      | to negative ID -> no massflow in the
      | pump (and no pressure drop calculations
      | necessary in the components of the
      | hydraulic loop)
  note: Unit delay to reduce
      | the max stepsize
  THBin : Inport
  Ctrl : Inport  Port=2
  Add : Sum  Inputs=3
  Add1 : Sum  Inputs=3
  Bus Assignment : BusAssignment  AssignedSignals=ID,Temperature,MassFlow,Pressure
  Bus Creator : BusCreator  Inputs=5
  Bus Selector : BusSelector  OutputSignals=ID,DPConstant,DPLinear,DPQuadratic
  Bus Selector1 : BusSelector  OutputSignals=DPQuadratic,DPLinear,DPConstant
  Constant : Constant
  Constant1 : Constant  Value=0:0.1:1.5
  Constant2 : Constant
  ElectricConsumptionPump : carnot/Basic/Hydraulics/ElectricConsumptionPump  e0=e0  e1=e1  e2=e2
      settings: SourceProductName=Carnot
  Gain{1..4} (4 alike) : Gain  Gain=-1
  Ground : Ground
  ID : Constant  Value=ID  mask{IDpreset=pressure drop}
      mask prompts: IDpreset "Calculation"
      mask init:
      | ID = IDpreset*10000 + 1;
      mask TypeOptions IDpreset: pressure drop | pressure drop and pressure head
  MATLAB Function : MATLAB Function  TreatAsAtomicUnit=on
  Memory : Memory
  Multiply{,1..3} (4 alike) : Product
  Mux2 : Mux  Inputs=7
  Pressure : Constant  Value=p0
  Pressuredrop : carnot/Basic/Pressure_Drop/Pressuredrop
      settings: SourceProductName=Carnot
  PumpHead : Gain  Gain=a0
  PumpLinear : Gain  Gain=a1
  PumpQuadratic : Constant  Value=a2
  S-Function : S-Function  FunctionName=pump  SFunctionDeploymentMode=off  EnableBusSupport=off
  Saturation : Saturate  UpperLimit=1  LowerLimit=0
  Square : Math  Operator=square  SaturateOnIntegerOverflow=on
  Square1 : Math  Operator=square  SaturateOnIntegerOverflow=on
  Switch1 : Switch  Criteria=u2 > Threshold  SaturateOnIntegerOverflow=on  InputSameDT=on
  Switch3 : Switch  Criteria=u2 > Threshold  SaturateOnIntegerOverflow=on  InputSameDT=on
  Terminator : Terminator
  Terminator1 : Terminator
  Terminator2 : Terminator
  ThermalNodeTHB : carnot/Basic/Thermal_Models/ThermalNodeTHB  UA=UA  mcp=mcp  Tini=Tini
      settings: SourceProductName=Carnot
  UnitDelay : UnitDelay  SampleTime=t1
  basic_THB : carnot/Basic/Hydraulics/basic_THB  t=20  mdot=0  p=p0  ID=No Pressure Drop  fluid=Water  mix=mix  mix2=mix2  mix3=mix3  dia=dia  hgt=0
      settings: SourceProductName=Carnot
  const5 : Constant  Value=0
  gain1 : Gain  Gain=-1  SaturateOnIntegerOverflow=on  OutDataTypeStr=Inherit: Same as input  ParamDataTypeStr=Inherit: Same as input
  THB : Outport
  Pdat : Outport  Port=2
  wires:
  ElectricConsumptionPump/1 -> Bus Creator/2  "PowerElectric"
  Bus Creator/1 -> Pdat/1  "Pdat"
  THBin/1 -> Bus Selector/1, ThermalNodeTHB/1, Bus Selector1/1
  Pressuredrop/3 -> Gain4/1
  Bus Selector/1 -> Switch1/2, Mux2/1  "<ID>"
  Switch1/1 -> Bus Assignment/4, ElectricConsumptionPump/1  "MassFlow"
  Mux2/1 -> S-Function/1
  S-Function/1 -> Memory/1
  Ctrl/1 -> Saturation/1, Bus Creator/5  "ControlSetpoint"
  ID/1 -> Switch3/1, gain1/1
  gain1/1 -> Switch3/3
  Memory/1 -> Pressuredrop/1, Switch1/1
  const5/1 -> Switch1/3
  basic_THB/1 -> Bus Assignment/1
  Bus Assignment/1 -> THB/1, Bus Creator/1  "THB"
  Switch3/1 -> Bus Assignment/2
  ThermalNodeTHB/1 -> Bus Assignment/3
  Bus Selector/2 -> Mux2/2  "<DPConstant>"
  Bus Selector/3 -> Mux2/3  "<DPLinear>"
  Bus Selector/4 -> Mux2/4  "<DPQuadratic>"
  Pressure/1 -> Pressuredrop/2
  Pressuredrop/1 -> Bus Assignment/5
  Ground/1 -> Pressuredrop/3
  Pressuredrop/2 -> Terminator/1
  Saturation/1 -> Switch3/2, PumpHead/1, ElectricConsumptionPump/2, Bus Creator/4  "ControlActual"
  Gain3/1 -> Pressuredrop/4
  Gain1/1 -> Pressuredrop/5
  Gain2/1 -> Pressuredrop/6
  Gain4/1 -> Bus Creator/3  "PumpHead"
  UnitDelay/1 -> Terminator1/1
  Constant/1 -> UnitDelay/1
  Square/1 -> Multiply/1
  Bus Selector1/3 -> Add/3  "<DPConstant>"
  Bus Selector1/2 -> Multiply1/2  "<DPLinear>"
  Bus Selector1/1 -> Multiply/2  "<DPQuadratic>"
  Multiply/1 -> Add/1
  Multiply1/1 -> Add/2
  Multiply3/1 -> Add1/2
  Multiply2/1 -> Add1/1
  PumpQuadratic/1 -> Gain2/1, Multiply2/2, Mux2/7  "<DPQuadratic>"
  PumpLinear/1 -> Gain1/1, Multiply3/2, Mux2/6  "<DPLinear>"
  PumpHead/1 -> Add1/3, Mux2/5, Gain3/1  "<DPConstant>"
  Square1/1 -> Multiply2/1
  Constant1/1 -> MATLAB Function/1(x), Multiply3/1, Square1/1, Multiply1/1, Square/1
  Add/1 -> MATLAB Function/2(y1)
  Add1/1 -> MATLAB Function/3(y2)
  MATLAB Function/1(y) -> Terminator2/1
  Constant2/1 -> PumpLinear/1

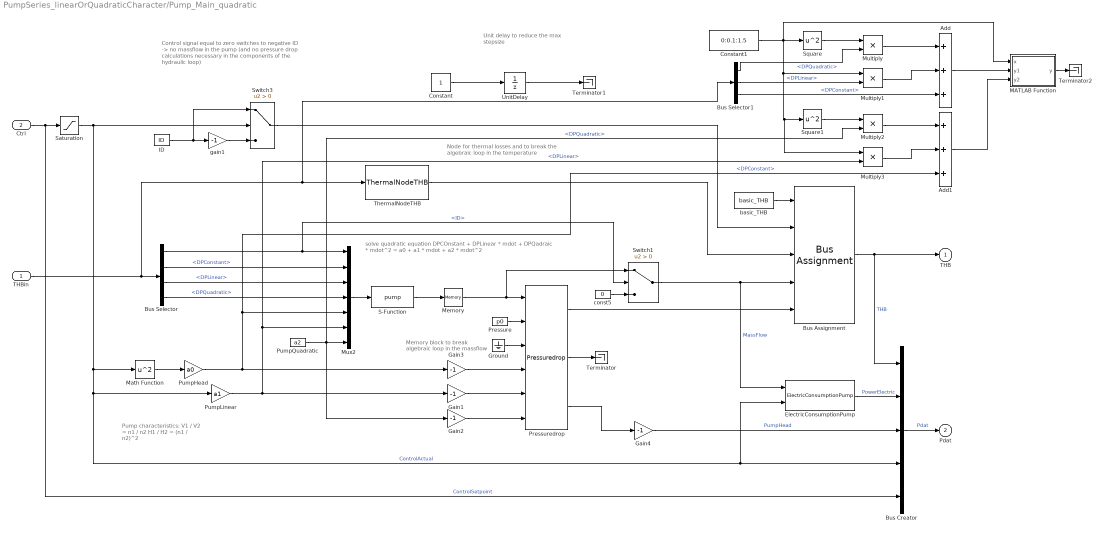
== system PumpSeries_linearOrQuadraticCharacter/Pump_Main_quadratic ==
  note: Unit delay to reduce
      | the max stepsize
  note: Pump characteristics:
      | V1 / V2 = n1 / n2
      | H1 / H2 = (n1 / n2)^2
  note: Control signal equal to zero switches
      | to negative ID -> no massflow in the
      | pump (and no pressure drop calculations
      | necessary in the components of the
      | hydraulic loop)
  note: solve quadratic equation
      | DPCOnstant + DPLinear * mdot + DPQadraic * mdot^2
      | = a0 + a1 * mdot + a2 * mdot^2
  note: Memory block to
      | break algebraic loop
      | in the massflow
  note: Node for thermal losses and to break
      | the algebraic loop in the temperature
  THBin : Inport
  Ctrl : Inport  Port=2
  Add : Sum  Inputs=3
  Add1 : Sum  Inputs=3
  Bus Assignment : BusAssignment  AssignedSignals=ID,Temperature,MassFlow,Pressure
  Bus Creator : BusCreator  Inputs=5
  Bus Selector : BusSelector  OutputSignals=ID,DPConstant,DPLinear,DPQuadratic
  Bus Selector1 : BusSelector  OutputSignals=DPQuadratic,DPLinear,DPConstant
  Constant : Constant
  Constant1 : Constant  Value=0:0.1:1.5
  ElectricConsumptionPump : carnot/Basic/Hydraulics/ElectricConsumptionPump  e0=e0  e1=e1  e2=e2
      settings: SourceProductName=Carnot
  Gain{1..4} (4 alike) : Gain  Gain=-1
  Ground : Ground
  ID : Constant  Value=ID  mask{IDpreset=pressure drop}
      mask prompts: IDpreset "Calculation"
      mask init:
      | ID = IDpreset*10000 + 1;
      mask TypeOptions IDpreset: pressure drop | pressure drop and pressure head
  MATLAB Function : MATLAB Function  TreatAsAtomicUnit=on
  Math Function : Math  Operator=square  SaturateOnIntegerOverflow=on
  Memory : Memory
  Multiply{,1..3} (4 alike) : Product
  Mux2 : Mux  Inputs=7
  Pressure : Constant  Value=p0
  Pressuredrop : carnot/Basic/Pressure_Drop/Pressuredrop
      settings: SourceProductName=Carnot
  PumpHead : Gain  Gain=a0
  PumpLinear : Gain  Gain=a1
  PumpQuadratic : Constant  Value=a2
  S-Function : S-Function  FunctionName=pump  SFunctionDeploymentMode=off  EnableBusSupport=off
  Saturation : Saturate  UpperLimit=1  LowerLimit=0
  Square : Math  Operator=square  SaturateOnIntegerOverflow=on
  Square1 : Math  Operator=square  SaturateOnIntegerOverflow=on
  Switch1 : Switch  Criteria=u2 > Threshold  SaturateOnIntegerOverflow=on  InputSameDT=on
  Switch3 : Switch  Criteria=u2 > Threshold  SaturateOnIntegerOverflow=on  InputSameDT=on
  Terminator : Terminator
  Terminator1 : Terminator
  Terminator2 : Terminator
  ThermalNodeTHB : carnot/Basic/Thermal_Models/ThermalNodeTHB  UA=UA  mcp=mcp  Tini=Tini
      settings: SourceProductName=Carnot
  UnitDelay : UnitDelay  SampleTime=t1
  basic_THB : carnot/Basic/Hydraulics/basic_THB  t=20  mdot=0  p=p0  ID=No Pressure Drop  fluid=Water  mix=mix  mix2=mix2  mix3=mix3  dia=dia  hgt=0
      settings: SourceProductName=Carnot
  const5 : Constant  Value=0
  gain1 : Gain  Gain=-1  SaturateOnIntegerOverflow=on  OutDataTypeStr=Inherit: Same as input  ParamDataTypeStr=Inherit: Same as input
  THB : Outport
  Pdat : Outport  Port=2
  wires:
  MATLAB Function/1(y) -> Terminator2/1
  Add1/1 -> MATLAB Function/3(y2)
  Add/1 -> MATLAB Function/2(y1)
  Constant1/1 -> Square/1, Multiply1/1, Square1/1, Multiply3/1, MATLAB Function/1(x)
  Square1/1 -> Multiply2/1
  PumpHead/1 -> Gain3/1, Mux2/5, Add1/3  "<DPConstant>"
  PumpLinear/1 -> Mux2/6, Multiply3/2, Gain1/1  "<DPLinear>"
  PumpQuadratic/1 -> Mux2/7, Multiply2/2, Gain2/1  "<DPQuadratic>"
  Multiply2/1 -> Add1/1
  Multiply3/1 -> Add1/2
  Multiply1/1 -> Add/2
  Multiply/1 -> Add/1
  Bus Selector1/1 -> Multiply/2  "<DPQuadratic>"
  Bus Selector1/2 -> Multiply1/2  "<DPLinear>"
  Bus Selector1/3 -> Add/3  "<DPConstant>"
  Square/1 -> Multiply/1
  Constant/1 -> UnitDelay/1
  UnitDelay/1 -> Terminator1/1
  Math Function/1 -> PumpHead/1
  Gain4/1 -> Bus Creator/3  "PumpHead"
  Gain2/1 -> Pressuredrop/6
  Gain1/1 -> Pressuredrop/5
  Gain3/1 -> Pressuredrop/4
  Saturation/1 -> Bus Creator/4, ElectricConsumptionPump/2, PumpLinear/1, Math Function/1, Switch3/2  "ControlActual"
  Pressuredrop/2 -> Terminator/1
  Ground/1 -> Pressuredrop/3
  Pressuredrop/1 -> Bus Assignment/5
  Pressure/1 -> Pressuredrop/2
  Bus Selector/4 -> Mux2/4  "<DPQuadratic>"
  Bus Selector/3 -> Mux2/3  "<DPLinear>"
  Bus Selector/2 -> Mux2/2  "<DPConstant>"
  ThermalNodeTHB/1 -> Bus Assignment/3
  Switch3/1 -> Bus Assignment/2
  Bus Assignment/1 -> Bus Creator/1, THB/1  "THB"
  basic_THB/1 -> Bus Assignment/1
  const5/1 -> Switch1/3
  Memory/1 -> Switch1/1, Pressuredrop/1
  gain1/1 -> Switch3/3
  ID/1 -> gain1/1, Switch3/1
  Ctrl/1 -> Bus Creator/5, Saturation/1  "ControlSetpoint"
  S-Function/1 -> Memory/1
  Mux2/1 -> S-Function/1
  Switch1/1 -> ElectricConsumptionPump/1, Bus Assignment/4  "MassFlow"
  Bus Selector/1 -> Mux2/1, Switch1/2  "<ID>"
  Pressuredrop/3 -> Gain4/1
  THBin/1 -> Bus Selector1/1, ThermalNodeTHB/1, Bus Selector/1
  Bus Creator/1 -> Pdat/1  "Pdat"
  ElectricConsumptionPump/1 -> Bus Creator/2  "PowerElectric"

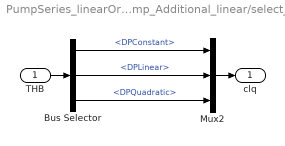
== system PumpSeries_linearOrQuadraticCharacter/Pump_Additional_linear/select_clq ==
  THB : Inport
  Bus Selector : BusSelector  OutputSignals=DPConstant,DPLinear,DPQuadratic
  Mux2 : Mux  Inputs=3
  clq : Outport
  wires:
  Bus Selector/3 -> Mux2/3  "<DPQuadratic>"
  Bus Selector/2 -> Mux2/2  "<DPLinear>"
  Bus Selector/1 -> Mux2/1  "<DPConstant>"
  THB/1 -> Bus Selector/1
  Mux2/1 -> clq/1

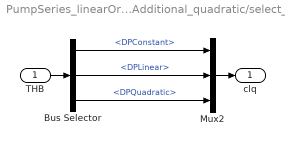
== system PumpSeries_linearOrQuadraticCharacter/Pump_Additional_quadratic/select_clq ==
  THB : Inport
  Bus Selector : BusSelector  OutputSignals=DPConstant,DPLinear,DPQuadratic
  Mux2 : Mux  Inputs=3
  clq : Outport
  wires:
  Mux2/1 -> clq/1
  THB/1 -> Bus Selector/1
  Bus Selector/1 -> Mux2/1  "<DPConstant>"
  Bus Selector/2 -> Mux2/2  "<DPLinear>"
  Bus Selector/3 -> Mux2/3  "<DPQuadratic>"

== matlab function PumpSeries_linearOrQuadraticCharacter/Pump_Main_quadratic/MATLAB Function ==
  data: x input; y output; y1 input; y2 input
function y = fcn(x, y1, y2)
figure(1)
plot(x,y1,x,y2)
title('Pump additional quadratic')
y = 0;

== matlab function PumpSeries_linearOrQuadraticCharacter/Pump_Main_linear/MATLAB Function ==
  data: x input; y output; y1 input; y2 input
function y = fcn(x, y1, y2)
figure(2)
plot(x,y1,x,y2)
title('Pump additional linear')
y = 0;
